simulink model "Overall_Mission"  (R2023a)
settings: Solver=VariableStepAuto  StartTime=0.0  StopTime=10.0  RelTol=1e-3
PreLoadFcn:
  | load AllBuses
settings Model: Creator=rose  LastModifiedBy=rose
settings OptimizationCC: DefaultParameterBehavior=Inlined

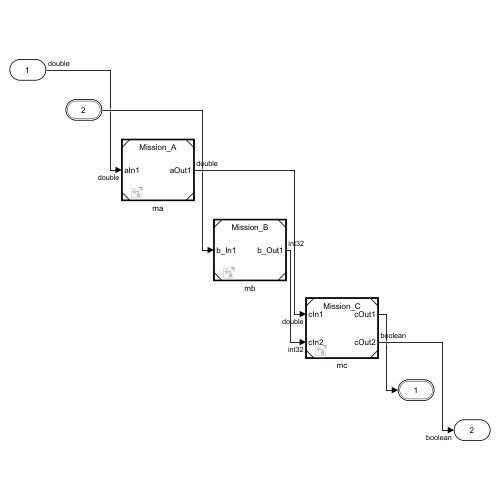
[thumbnail: Simulink's stored preview of the top-level diagram]
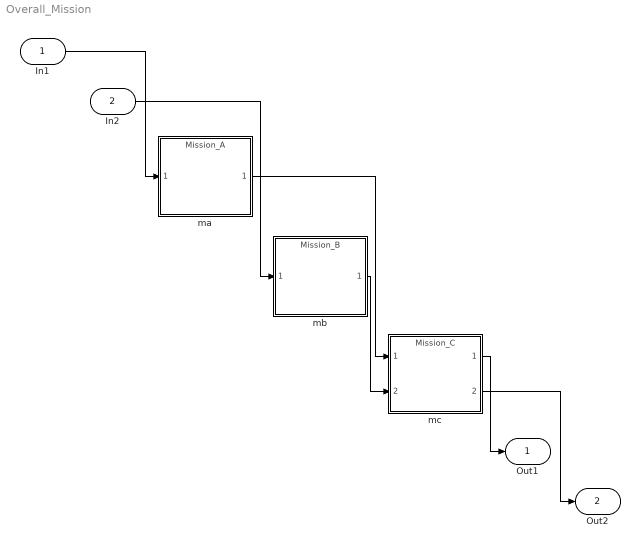
== system Overall_Mission ==
  In1 : Inport  OutDataTypeStr=double
  In2 : Inport  Port=2  OutDataTypeStr=Bus: Bus_2  BusOutputAsStruct=on
  ma : ModelReference  ModelNameDialog=Mission_A  SimulationMode=Normal  ModelReferenceVersion=1.1
  mb : ModelReference  ModelNameDialog=Mission_B  SimulationMode=Normal  ModelReferenceVersion=1.1
  mc : ModelReference  ModelNameDialog=Mission_C  SimulationMode=Normal  ModelReferenceVersion=1.1
  Out1 : Outport  OutDataTypeStr=Bus: Bus_1  BusOutputAsStruct=on
  Out2 : Outport  Port=2  OutDataTypeStr=boolean
  wires:
  In1/1 -> ma/1
  In2/1 -> mb/1
  ma/1 -> mc/1
  mb/1 -> mc/2
  mc/1 -> Out1/1
  mc/2 -> Out2/1
